simulink model "exemplo_filtro_media_movel_2"  (R2019b)
settings: Solver=VariableStepAuto  StartTime=0.0  StopTime=0.075  RelTol=1e-3
values from neighbouring files (symbols this model uses):
  T = 0.00833333333333    [ECG_graficos_fft.mat]    (also in FPB_Arduino.mat = 0.001; butter1.mat = 1.25e-08; filtro_notch1.mat; intro_resp_freq.mat = 0.00125)
settings Model: Creator=fernandopassold  LastModifiedBy=fernandopassold

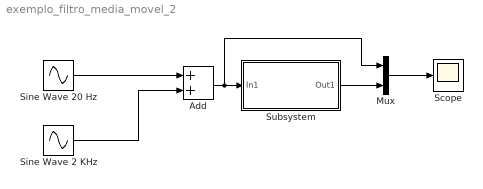
== system exemplo_filtro_media_movel_2 ==
  Add : Sum
  Mux : Mux  Inputs=2
  Scope : Scope
  Sine Wave 2 KHz : Sin  Amplitude=0.1  Frequency=2*pi*2000  SampleTime=0
  Sine Wave 20 Hz : Sin  Frequency=2*pi*20  SampleTime=0
  Subsystem : Subsystem
  wires:
  Add/1 -> Mux/1, Subsystem/1(In1)
  Sine Wave 20 Hz/1 -> Add/1
  Sine Wave 2 KHz/1 -> Add/2
  Subsystem/1(Out1) -> Mux/2
  Mux/1 -> Scope/1

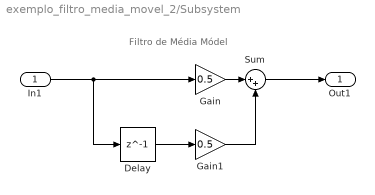
== system exemplo_filtro_media_movel_2/Subsystem ==
  note: Filtro de Média Módel
  In1 : Inport
  Delay : Delay  DelayLength=1  SampleTime=T
  Gain : Gain  Gain=0.5
  Gain1 : Gain  Gain=0.5
  Sum : Sum  Inputs=|++
  Out1 : Outport
  wires:
  Sum/1 -> Out1/1
  Gain/1 -> Sum/1
  Gain1/1 -> Sum/2
  In1/1 -> Delay/1, Gain/1
  Delay/1 -> Gain1/1
